simulink model "CoETS_TSEACo"  (R2016b)
settings: configuration reference "CodeGenConfigSet" (kept outside this file)
values from neighbouring files (symbols this model uses):
  CoETS_ctEngEmgcyRunCnt_C = Calibration.Parameter    [init_CoETS_TSEACo.m]
  CoETS_nTSCRmpSlopeNeg_C = Calibration.Parameter    [init_CoETS_TSEACo.m]
  CoETS_nTSCRmpSlopePos_C = Calibration.Parameter    [init_CoETS_TSEACo.m]
  CoETS_numTSEAPrioAE_C = Calibration.Parameter    [init_CoETS_TSEACo.m]
  CoETS_numTSEAPrioDE_C = Calibration.Parameter    [init_CoETS_TSEACo.m]
  CoETS_numTSEAPrioGpsLim_C = Calibration.Parameter    [init_CoETS_TSEACo.m]
  CoETS_numTSEAPrioPE_C = Calibration.Parameter    [init_CoETS_TSEACo.m]
  CoETS_numTSEAPrioTE_C = Calibration.Parameter    [init_CoETS_TSEACo.m]
  CoETS_numTSEAPrioVE_C = Calibration.Parameter    [init_CoETS_TSEACo.m]
  CoETS_stEngEmgcyRunEN_C = Calibration.Parameter    [init_CoETS_TSEACo.m]
  CoETS_stStartRelayCtrl_C = Calibration.Parameter    [init_CoETS_TSEACo.m]
  CoETS_stTboxUse_C = Calibration.Parameter    [init_CoETS_TSEACo.m]
  CoETS_stTSEATrqSpd_C = Calibration.Parameter    [init_CoETS_TSEACo.m]
  CoETS_swtTempSel_C = Calibration.Parameter    [init_CoETS_TSEACo.m]
  CoETS_tEngEmgcyRunTemp_C = Calibration.Parameter    [init_CoETS_TSEACo.m]
  CoETS_tiEngEmgcyRunTime_C = Calibration.Parameter    [init_CoETS_TSEACo.m]
  CoETS_tiEngEmgcyStartTime_C = Calibration.Parameter    [init_CoETS_TSEACo.m]
  CoETS_tiEngLockTime_C = Calibration.Parameter    [init_CoETS_TSEACo.m]
  CoETS_tiSetTimeTSEReq_CUR = Calibration.Parameter    [init_CoETS_TSEACo.m]
  CoETS_tiSetTimeTSEReq_CURX = Calibration.Parameter    [init_CoETS_TSEACo.m]
  CoETS_TrqTSCRmpSlopeNeg_C = Calibration.Parameter    [init_CoETS_TSEACo.m]
  CoETS_TrqTSCRmpSlopePos_C = Calibration.Parameter    [init_CoETS_TSEACo.m]
  Ecu_stGps_Status_C = Calibration.Parameter    [init_CoETS_TSEACo.m]
  EngPrt_nRateSp_C = Calibration.Parameter    [init_CoETS_TSEACo.m]
  Gps_nSpdLmt_C = Calibration.Parameter    [init_CoETS_TSEACo.m]
  TSC_nAEDes_C = Calibration.Parameter    [init_CoETS_TSEACo.m]
  TSC_nDEDes_C = Calibration.Parameter    [init_CoETS_TSEACo.m]
  TSC_nPEDes_C = Calibration.Parameter    [init_CoETS_TSEACo.m]
  TSC_nTEDes_C = Calibration.Parameter    [init_CoETS_TSEACo.m]
  TSC_nVEDes_C = Calibration.Parameter    [init_CoETS_TSEACo.m]
  TSC_rTrqAEDes_C = Calibration.Parameter    [init_CoETS_TSEACo.m]
  TSC_rTrqDEDes_C = Calibration.Parameter    [init_CoETS_TSEACo.m]
  TSC_rTrqPEDes_C = Calibration.Parameter    [init_CoETS_TSEACo.m]
  TSC_rTrqTEDes_C = Calibration.Parameter    [init_CoETS_TSEACo.m]
  TSC_rTrqVEDes_C = Calibration.Parameter    [init_CoETS_TSEACo.m]
  TSC_stAEErr_C = Calibration.Parameter    [init_CoETS_TSEACo.m]
  TSC_stAEMode_C = Calibration.Parameter    [init_CoETS_TSEACo.m]
  TSC_stDEErr_C = Calibration.Parameter    [init_CoETS_TSEACo.m]
  TSC_stDEMode_C = Calibration.Parameter    [init_CoETS_TSEACo.m]
  TSC_stModeBypassEN_C = Calibration.Parameter    [init_CoETS_TSEACo.m]
  TSC_stPEErr_C = Calibration.Parameter    [init_CoETS_TSEACo.m]
  TSC_stPEMode_C = Calibration.Parameter    [init_CoETS_TSEACo.m]
  TSC_stTEErr_C = Calibration.Parameter    [init_CoETS_TSEACo.m]
  TSC_stTEMode_C = Calibration.Parameter    [init_CoETS_TSEACo.m]
  TSC_stVEErr_C = Calibration.Parameter    [init_CoETS_TSEACo.m]
  TSC_stVEMode_C = Calibration.Parameter    [init_CoETS_TSEACo.m]
undefined symbols (not defined in the file or in its folder): CoETS_TSEACo_DT, EngState_conv, HLSDem_KpCorFac_MAPX, Switch_conv, TSC1_stSource_conv
libraries: simulink x82, CXLib x8
(part 2 of 2)

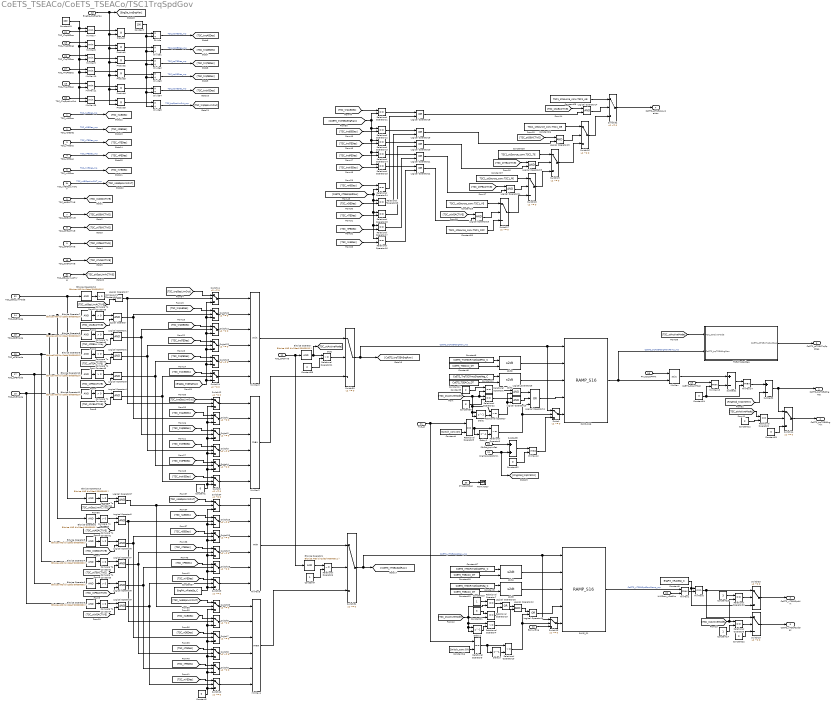
== system CoETS_TSEACo/CoETS_TSEACo/TSC1TrqSpdGov ==
  TSC_nAEDes : Inport  Tag=rpm  Description=Requested speed / speed limit by TSC1-AE message  OutMin=0  OutMax=6000  OutDataTypeStr=EngSpeed_rpm
  TSC_nDEDes : Inport  Tag=rpm  Description=|  Port=2  OutMin=0  OutMax=8000  OutDataTypeStr=EngSpeed_rpm
      | Requested speed / speed limit by TSC1-DE CAN
      | message rpm
  TSC_nTEDes : Inport  Tag=rpm  Description=|  Port=3  OutMin=0  OutMax=8000  OutDataTypeStr=EngSpeed_rpm
      | Requested speed / speed limit by TSC1-TE CAN
      | message rpm
  TSC_nPEDes : Inport  Tag=rpm  Description=|  Port=4  OutMin=0  OutMax=8000  OutDataTypeStr=EngSpeed_rpm
      | Requested speed / speed limit by TSC1-PE CAN
      | message rpm
  TSC_nVEDes : Inport  Tag=rpm  Description=|  Port=5  OutMin=0  OutMax=8000  OutDataTypeStr=EngSpeed_rpm
      | Requested speed / speed limit by TSC1-VE CAN
      | message rpm
  TSC_stAEACTIVE : Inport  Port=6
  TSC_stDEACTIVE : Inport  Port=7
  TSC_stTEACTIVE : Inport  Port=8
  TSC_stPEACTIVE : Inport  Port=9
  TSC_stVEACTIVE : Inport  Port=10
  TSC_stACTIVE : Inport  Port=11
  Epm_nEng : Inport  Tag=rpm  Description=Engine speed  Port=12  OutMin=0  OutMax=6000  OutDataTypeStr=EngSpeed_rpm
  PT_trqCrSPTPrt : Inport  Tag=Nm  Description=Application parameter for powertrain protection train protection torque(crankshaft torque)  Port=13  OutMin=-3000  OutMax=3000  OutDataTypeStr=Trq_Nm
  TSC_stAEMode : Inport  Description=Override control mode of TSC1-AE CAN message  Port=14  OutMin=0  OutMax=3  OutDataTypeStr=State_uint8
  TSC_stDEMode : Inport  Description=Override control mode of TSC1-DE CAN message  Port=15  OutMin=0  OutMax=3  OutDataTypeStr=State_uint8
  TSC_stTEMode : Inport  Description=Override control mode of TSC1-TE CAN message  Port=16  OutMin=0  OutMax=3  OutDataTypeStr=State_uint8
  TSC_stPEMode : Inport  Description=Override control mode of TSC1-PE CAN message  Port=17  OutMin=0  OutMax=3  OutDataTypeStr=State_uint8
  TSC_stVEMode : Inport  Description=Override control mode of TSC1-VE CAN message.  Port=18  OutMin=0  OutMax=3  OutDataTypeStr=State_uint8
  PthSet_trqInrSet : Inport  Port=19
  HLSDem_nSetPLo : Inport  Port=20
  T15_st : Inport  Port=21
  RngMod_trqCrSMin : Inport  Port=22
  EngDa_trqEngMax : Inport  Tag=Nm  Description=Maximum engine output torque  Port=23  OutMin=-3276.8  OutMax=3276.7  OutDataTypeStr=Trq_Nm
  TSC_rTrqAEDes : Inport  Description=|  Port=24  OutMin=0  OutMax=125  OutDataTypeStr=State_uint8
      | Requested torque percent / torque limit by TSC1-AE CAN
      | message Nm
  TSC_rTrqDEDes : Inport  Description=|  Port=25  OutMin=0  OutMax=125  OutDataTypeStr=State_uint8
      | Requested torque percent/ torque limit by TSC1-DE CAN
      | message Nm
  TSC_rTrqTEDes : Inport  Description=|  Port=26  OutMin=0  OutMax=125  OutDataTypeStr=State_uint8
      | Requested torque percent / torque limit by TSC1-TE CAN
      | message Nm
  TSC_rTrqPEDes : Inport  Description=|  Port=27  OutMin=0  OutMax=125  OutDataTypeStr=State_uint8
      | Requested torque percent/ torque limit by TSC1-PE CAN
      | message Nm
  TSC_rTrqVEDes : Inport  Description=|  Port=28  OutMin=0  OutMax=125  OutDataTypeStr=State_uint8
      | Requested torque percent/ torque limit by TSC1-VE CAN
      | message Nm
  CoETS_trqUnFltLtd : Inport  Port=29
  PT_trqCrSDes : Inport  Tag=Nm  Description=Application parameter for requested propulsion torque to engine(crankshaft torque)  Port=30
  TSC_stGpsLimACTIVE : Inport  Port=31
  TSC_stGpsLimMode : Inport  Description=Override control mode of TSC1-AE CAN message  Port=32  OutMin=0  OutMax=3  OutDataTypeStr=State_uint8
  TSC_rTrqGpsLimOut : Inport  Description=|  Port=33  OutMin=0  OutMax=125  OutDataTypeStr=State_uint8
      | Requested torque percent/ torque limit by TSC1-VE CAN
      | message Nm
  TSC_nAEGpsLimOUT : Inport  Tag=rpm  Description=Requested speed / speed limit by TSC1-AE message  Port=34  OutMin=0  OutMax=6000  OutDataTypeStr=EngSpeed_rpm
  Bitwise Operator : simulink/Logic and Bit Operations/Bitwise Operator  logicop=AND  UseBitMask=on  BitMask=bin2dec('00000011')  BitMaskRealWorld=Stored Integer
  Bitwise Operator1 : simulink/Logic and Bit Operations/Bitwise Operator  logicop=AND  UseBitMask=on  BitMask=bin2dec('00000011')  BitMaskRealWorld=Stored Integer
  Bitwise Operator{7..12} (6 alike) : simulink/Logic and Bit Operations/Bitwise Operator  logicop=AND  UseBitMask=on  BitMask=bin2dec('00000010')  BitMaskRealWorld=Stored Integer
  Bitwise Operator{2..6,13} (6 alike) : simulink/Logic and Bit Operations/Bitwise Operator  logicop=AND  UseBitMask=on  BitMask=bin2dec('00000001')  BitMaskRealWorld=Stored Integer
  Compare To Constant{,1..11} (12 alike) : simulink/Logic and Bit Operations/Compare To Constant  relop=>  const=0  OutDataTypeStr=boolean
  Constant : Constant  Value=100  OutDataTypeStr=Inherit: Inherit via back propagation
  Constant{1..2,22,24,31..32} (6 alike) : Constant  Value=0  OutDataTypeStr=Inherit: Inherit via back propagation
  Constant10 : Constant  Value=CoETS_TrqTSCRmpSlopeNeg_C
  Constant{8,11,13,18} (4 alike) : Constant  Value=CoETS_TSEACo_DT
  Constant12 : Constant  Value=2  OutDataTypeStr=Inherit: Inherit via back propagation
  Constant14 : Constant  OutDataTypeStr=Inherit: Inherit via back propagation
  Constant15 : Constant  OutDataTypeStr=Inherit: Inherit via back propagation
  Constant16 : Constant  Value=Switch_conv.ON
  Constant17 : Constant  Value=CoETS_nTSCRmpSlopePos_C
  Constant19 : Constant  Value=100  OutDataTypeStr=Inherit: Inherit via back propagation
  Constant20 : Constant  Value=TSC1_stSource_conv.TSC1_OFF
  Constant21 : Constant  Value=3  OutDataTypeStr=Inherit: Inherit via back propagation
  Constant23 : Constant  Value=3  OutDataTypeStr=Inherit: Inherit via back propagation
  Constant25 : Constant  Value=TSC1_stSource_conv.TSC1_AE
  Constant26 : Constant  Value=TSC1_stSource_conv.TSC1_DE
  Constant27 : Constant  Value=TSC1_stSource_conv.TSC1_PE
  Constant28 : Constant  Value=TSC1_stSource_conv.TSC1_TE
  Constant29 : Constant  Value=TSC1_stSource_conv.TSC1_VE
  Constant3 : Constant  Value=2  OutDataTypeStr=Inherit: Inherit via back propagation
  Constant30 : Constant  Value=3  OutDataTypeStr=Inherit: Inherit via back propagation
  Constant37 : Constant  Value=EngPrt_nRateSp_C
  Constant38 : Constant  Value=2  OutDataTypeStr=Inherit: Inherit via back propagation
  Constant4 : Constant  Value=Switch_conv.ON
  Constant5 : Constant  Value=CoETS_nTSCRmpSlopeNeg_C
  Constant6 : Constant  Value=CoETS_TrqTSCRmpSlopePos_C
  Constant7 : Constant  OutDataTypeStr=Inherit: Inherit via back propagation
  Constant9 : Constant  Value=EngPrt_nRateSp_C
  Delay : Delay  DelayLength=1  InitialConditionSource=Input port  InitialCondition=0
      settings: InputPortMap=u0,p4
  Delay1 : Delay  DelayLength=1  InitialCondition=0
  Delay2 : Delay  DelayLength=1  InitialConditionSource=Input port  InitialCondition=0
      settings: InputPortMap=u0,p4
  Delay3 : Delay  DelayLength=1  InitialCondition=0
  Divide{,1..5} (6 alike) : Product  Inputs=*/  OutDataTypeStr=Inherit: Inherit via back propagation  SaturateOnIntegerOverflow=on
  Logical Operator{,1..10,12,14..15,17,23..27} (20 alike) : Logic  AllPortsSameDT=off  OutDataTypeStr=boolean
  Logical Operator11 : Logic  Operator=OR  Inputs=3  AllPortsSameDT=off  OutDataTypeStr=boolean
  Logical Operator{13,16,18..22} (7 alike) : Logic  Operator=OR  AllPortsSameDT=off  OutDataTypeStr=boolean
  MinMax{,6..11,15} (8 alike) : MinMax  Inputs=2
  MinMax{1,12..14} (4 alike) : MinMax  Function=max  Inputs=2
  MinMax2 : MinMax  Function=max  Inputs=6
  MinMax3 : MinMax  Inputs=6
  MinMax4 : MinMax  Function=max  Inputs=6
  MinMax5 : MinMax  Inputs=6
  Product{,1..5} (6 alike) : Product  SaturateOnIntegerOverflow=on
  RAMP_S1 : CXLib/RAMP_S16
  RAMP_S16 : CXLib/RAMP_S16
  Relational Operator{,4..6,10,21} (6 alike) : RelationalOperator  Operator=~=  OutDataTypeStr=boolean  RndMeth=Simplest
  Relational Operator{1..3,7..9,11..20,22..24} (19 alike) : RelationalOperator  Operator===  OutDataTypeStr=boolean  RndMeth=Simplest
  Subtract1 : Sum  Inputs=+-  OutDataTypeStr=Inherit: Inherit via back propagation  SaturateOnIntegerOverflow=on  InputSameDT=on
  Subtract2 : Sum  Inputs=+-  OutDataTypeStr=Inherit: Inherit via back propagation  SaturateOnIntegerOverflow=on  InputSameDT=on
  Subtract3 : Sum  OutDataTypeStr=Inherit: Inherit via back propagation  SaturateOnIntegerOverflow=on  InputSameDT=on
  Switch{,1..35} (36 alike) : Switch  Criteria=u2 ~= 0
  TSEATrqSpdReq : Subsystem
  Terminator : Terminator
  s2dt{1..4} (4 alike) : CXLib/s2dt
  CoETS_trqTSEAEngMax : Outport
  CoETS_trqTSEAEngMin : Outport  Tag=Nm  Description=torque request to engine intervention increment(Min)  Port=2  OutMin=-3276  OutMax=3276  OutDataTypeStr=Trq_Nm
  CoETS_nTSEASpdLim : Outport  Port=3
  CoETS_stTSEASourceActv : Outport  Description=Identification name / number of the currently active EISGov client, which determines the current controller parameters  Port=4
  CoETS_nTSEASpdDes : Outport  Port=5
  CoETS_stTSEATrqSpdReq : Outport  Port=6
  wires:
  Switch30/1 -> [CoETS_trqTSEAEngRaw], RAMP_S16/1, Switch/1  "CoETS_trqTSEAEngRaw_mp"
  MinMax3/1 -> Switch30/1
  MinMax2/1 -> Switch30/3
  Constant38/1 -> Relational Operator21/2
  MinMax4/1 -> Switch31/3
  MinMax5/1 -> Switch31/1
  Relational Operator21/1 -> Switch30/2
  Bitwise Operator/1 -> Relational Operator21/1, [TSC_stActiveMode]
  [EngDa_trqEngMax] -> Switch11/3, Switch20/3, Switch21/3, Switch22/3, Switch23/3, Switch24/3
  Constant37/1 -> Switch25/3, Switch34/3, Switch26/3, Switch27/3, Switch28/3, Switch29/3
  Constant1/1 -> Switch4/3, Switch3/3, Switch2/3, Switch1/3, Switch12/3, Switch5/3
  Constant2/1 -> Switch35/3, Switch6/3, Switch7/3, Switch8/3, Switch9/3, Switch10/3
  Constant7/1 -> Relational Operator6/2
  Bitwise Operator1/1 -> Relational Operator6/1
  Relational Operator6/1 -> Switch31/2
  [TSC_stActiveMode] -> Relational Operator1/2, Relational Operator22/1, Relational Operator/1, Delay/2, Delay/1
  Delay/1 -> Relational Operator/2
  Compare To Constant5/1 -> Logical Operator/1
  TSC_stAEACTIVE/1 -> [TSC_stAEACTIVE]
  Compare To Constant6/1 -> Logical Operator1/1
  Compare To Constant7/1 -> Logical Operator2/1
  Logical Operator1/1 -> Switch2/2, Switch21/2
  Logical Operator2/1 -> Switch3/2, Switch22/2
  Compare To Constant8/1 -> Logical Operator3/1
  Logical Operator3/1 -> Switch4/2, Switch23/2
  Compare To Constant9/1 -> Logical Operator4/1
  Logical Operator4/1 -> Switch5/2, Switch24/2
  Logical Operator/1 -> Switch20/2, Switch1/2
  TSC_stAEMode/1 -> Bitwise Operator7/1, Bitwise Operator2/1
  Bitwise Operator2/1 -> Compare To Constant/1
  Bitwise Operator3/1 -> Compare To Constant1/1
  TSC_stDEMode/1 -> Bitwise Operator8/1, Bitwise Operator3/1
  Bitwise Operator4/1 -> Compare To Constant2/1
  TSC_stTEMode/1 -> Bitwise Operator9/1, Bitwise Operator4/1
  Bitwise Operator5/1 -> Compare To Constant3/1
  TSC_stPEMode/1 -> Bitwise Operator10/1, Bitwise Operator5/1
  Bitwise Operator6/1 -> Compare To Constant4/1
  TSC_stVEMode/1 -> Bitwise Operator11/1, Bitwise Operator6/1
  Bitwise Operator7/1 -> Compare To Constant5/1
  Bitwise Operator8/1 -> Compare To Constant6/1
  Bitwise Operator9/1 -> Compare To Constant7/1
  Bitwise Operator10/1 -> Compare To Constant8/1
  Bitwise Operator11/1 -> Compare To Constant9/1
  Compare To Constant/1 -> Logical Operator5/1
  TSC_stDEACTIVE/1 -> [TSC_stDEACTIVE]
  TSC_stTEACTIVE/1 -> [TSC_stTEACTIVE]
  TSC_stPEACTIVE/1 -> [TSC_stPEACTIVE]
  TSC_stVEACTIVE/1 -> [TSC_stVEACTIVE]
  [TSC_stAEACTIVE] -> Logical Operator/2
  [TSC_stDEACTIVE] -> Logical Operator1/2
  [TSC_stTEACTIVE] -> Logical Operator2/2
  [TSC_stPEACTIVE] -> Logical Operator3/2
  [TSC_stVEACTIVE] -> Logical Operator4/2
  [TSC_stAEACTIVE] -> Logical Operator5/2
  Logical Operator5/1 -> Switch6/2, Switch25/2
  Compare To Constant1/1 -> Logical Operator6/1
  [TSC_stDEACTIVE] -> Logical Operator6/2
  Logical Operator6/1 -> Switch7/2, Switch26/2
  Compare To Constant2/1 -> Logical Operator7/1
  [TSC_stTEACTIVE] -> Logical Operator7/2
  Compare To Constant3/1 -> Logical Operator8/1
  [TSC_stPEACTIVE] -> Logical Operator8/2
  Compare To Constant4/1 -> Logical Operator9/1
  [TSC_stVEACTIVE] -> Logical Operator9/2
  Logical Operator7/1 -> Switch8/2, Switch27/2
  Logical Operator8/1 -> Switch9/2, Switch28/2
  Logical Operator9/1 -> Switch10/2, Switch29/2
  Constant3/1 -> Relational Operator1/1
  Relational Operator/1 -> Logical Operator10/2, Logical Operator26/2
  RAMP_S16/1 -> TSEATrqSpdReq/2(CoETS_trqTSEAEngRaw), MinMax/2  "CoETS_trqTSEAEngRawRamp_mp"
  Constant8/1 -> s2dt2/2
  Constant6/1 -> s2dt2/1
  s2dt2/1 -> RAMP_S16/2
  Constant11/1 -> s2dt1/2
  Constant10/1 -> s2dt1/1
  s2dt1/1 -> RAMP_S16/3
  Switch14/1 -> CoETS_trqTSEAEngMin/1
  [TSC_stActiveMode] -> Relational Operator2/1
  Constant12/1 -> Relational Operator2/2
  Relational Operator2/1 -> Switch14/2
  Switch/1 -> RAMP_S16/5
  Logical Operator11/1 -> RAMP_S16/4
  Constant4/1 -> Relational Operator3/2
  Delay1/1 -> Relational Operator5/2
  Relational Operator3/1 -> Delay1/1, Relational Operator5/1
  Relational Operator5/1 -> Logical Operator11/3, Switch/2
  PT_trqCrSPTPrt/1 -> MinMax/1
  [TSC_stActiveMode] -> Relational Operator19/2, Delay2/2, Delay2/1, Relational Operator4/1, Relational Operator7/2
  Delay2/1 -> Relational Operator4/2
  Constant15/1 -> Relational Operator7/1
  Relational Operator4/1 -> Logical Operator12/2
  MinMax6/1 -> Switch33/1, Switch15/1
  Constant18/1 -> s2dt4/2
  Constant17/1 -> s2dt4/1
  s2dt4/1 -> RAMP_S1/2
  Constant13/1 -> s2dt3/2
  Constant5/1 -> s2dt3/1
  s2dt3/1 -> RAMP_S1/3
  Constant14/1 -> Relational Operator8/2
  Relational Operator8/1 -> Switch15/2
  Epm_nEng/1 -> Switch13/3
  Switch13/1 -> RAMP_S1/5
  Logical Operator12/1 -> Logical Operator13/1
  Logical Operator13/1 -> RAMP_S1/4
  T15_st/1 -> Relational Operator3/1, Relational Operator9/1
  Constant16/1 -> Relational Operator9/2
  Delay3/1 -> Relational Operator10/2
  Relational Operator9/1 -> Delay3/1, Relational Operator10/1
  Relational Operator10/1 -> Switch13/2, Logical Operator13/2
  Constant22/1 -> Switch15/3
  Constant25/1 -> Switch32/1
  Constant27/1 -> Switch18/1
  Constant28/1 -> Switch19/1
  Constant26/1 -> Switch16/1
  Constant20/1 -> Switch17/3
  Constant29/1 -> Switch17/1
  Switch17/1 -> Switch18/3
  Switch18/1 -> Switch19/3
  Switch19/1 -> Switch16/3
  Switch16/1 -> Switch32/3
  Switch32/1 -> CoETS_stTSEASourceActv/1
  [TSC_stAEACTIVE] -> Logical Operator14/1
  TSC_nAEDes/1 -> [TSC_nAEDes]  "TSC_nAEDes_mp"
  TSC_nDEDes/1 -> [TSC_nDEDes]  "TSC_nDEDes_mp"
  TSC_nTEDes/1 -> [TSC_nTEDes]  "TSC_nTEDes_mp"
  TSC_nPEDes/1 -> [TSC_nPEDes]  "TSC_nPEDes_mp"
  TSC_nVEDes/1 -> [TSC_nVEDes]  "TSC_nVEDes_mp"
  [TSC_trqAEDes] -> Switch20/1
  [TSC_trqAEDes] -> Switch1/1
  [TSC_trqDEDes] -> Switch21/1
  [TSC_trqDEDes] -> Switch2/1
  [TSC_trqTEDes] -> Switch22/1
  [TSC_trqTEDes] -> Switch3/1
  [TSC_trqPEDes] -> Switch23/1
  [TSC_trqPEDes] -> Switch4/1
  [TSC_trqVEDes] -> Switch24/1
  [TSC_trqVEDes] -> Switch5/1
  [TSC_nAEDes] -> Switch25/1
  [TSC_nAEDes] -> Switch6/1
  [TSC_nDEDes] -> Switch7/1
  [TSC_nDEDes] -> Switch26/1
  [TSC_nTEDes] -> Switch27/1
  [TSC_nTEDes] -> Switch8/1
  [TSC_nPEDes] -> Switch9/1
  [TSC_nVEDes] -> Switch10/1
  [TSC_nVEDes] -> Switch29/1
  [TSC_nPEDes] -> Switch28/1
  Logical Operator14/1 -> Switch32/2
  [TSC_stDEACTIVE] -> Logical Operator15/1
  [TSC_trqDEDes] -> Relational Operator12/2
  Logical Operator15/1 -> Switch16/2
  [TSC_trqAEDes] -> Relational Operator11/1
  [CoETS_trqTSEAEngRaw] -> Relational Operator11/2, Relational Operator15/1, Relational Operator14/1, Relational Operator13/1, Relational Operator12/1
  [TSC_trqTEDes] -> Relational Operator13/2
  [TSC_trqPEDes] -> Relational Operator14/2
  [TSC_trqVEDes] -> Relational Operator15/2
  Switch31/1 -> [CoETS_nTSEASpdRaw], RAMP_S1/1, Switch13/1  "CoETS_nTSEASpdRaw_mp"
  [TSC_nVEDes] -> Relational Operator16/2
  [TSC_nPEDes] -> Relational Operator17/2
  Constant21/1 -> Relational Operator19/1
  Relational Operator7/1 -> Logical Operator16/1
  Relational Operator19/1 -> Logical Operator16/2
  Logical Operator16/1 -> Logical Operator12/1
  Switch15/1 -> CoETS_nTSEASpdDes/1
  Switch33/1 -> CoETS_nTSEASpdLim/1
  [TSC_stActiveMode] -> Relational Operator20/2, Relational Operator8/1
  Relational Operator20/1 -> Switch33/2
  Constant23/1 -> Relational Operator20/1
  Constant30/1 -> Relational Operator22/2
  Constant31/1 -> Switch14/3
  [TSC_nTEDes] -> Relational Operator18/2
  Constant9/1 -> Switch33/3, MinMax6/1
  [TSC_nDEDes] -> Relational Operator23/2
  [TSC_nAEDes] -> Relational Operator24/1
  [CoETS_nTSEASpdRaw] -> Relational Operator16/1, Relational Operator17/1, Relational Operator18/1, Relational Operator23/1, Relational Operator24/2
  Relational Operator11/1 -> Logical Operator18/1
  Relational Operator24/1 -> Logical Operator18/2
  Relational Operator12/1 -> Logical Operator19/1
  Relational Operator23/1 -> Logical Operator19/2
  Relational Operator13/1 -> Logical Operator20/1
  Relational Operator18/1 -> Logical Operator20/2
  Relational Operator14/1 -> Logical Operator21/1
  Relational Operator17/1 -> Logical Operator21/2
  Relational Operator15/1 -> Logical Operator22/1
  Relational Operator16/1 -> Logical Operator22/2
  Logical Operator18/1 -> Logical Operator14/2
  Logical Operator19/1 -> Logical Operator15/2
  [TSC_stTEACTIVE] -> Logical Operator23/1
  Logical Operator23/1 -> Switch19/2
  Logical Operator20/1 -> Logical Operator23/2
  [TSC_stPEACTIVE] -> Logical Operator24/1
  Logical Operator24/1 -> Switch18/2
  Logical Operator21/1 -> Logical Operator24/2
  [TSC_stVEACTIVE] -> Logical Operator25/1
  Logical Operator25/1 -> Switch17/2
  Logical Operator22/1 -> Logical Operator25/2
  HLSDem_nSetPLo/1 -> MinMax1/2
  RAMP_S1/1 -> MinMax1/1  "CoETS_nTSEASpdRawRamp_mp"
  MinMax1/1 -> MinMax6/2
  EngDa_trqEngMax/1 -> Product5/2, Product4/2, Product3/2, Product2/2, Product1/2, Product/2, [EngDa_trqEngMax]
  Divide/1 -> [TSC_trqAEDes]  "TSC_trqAEDes_mp"
  Product1/1 -> Divide1/1
  Product/1 -> Divide/1
  Divide1/1 -> [TSC_trqDEDes]  "TSC_trqDEDes_mp"
  Product2/1 -> Divide2/1
  Divide2/1 -> [TSC_trqTEDes]  "TSC_trqTEDes_mp"
  Product3/1 -> Divide3/1
  Divide3/1 -> [TSC_trqPEDes]  "TSC_trqPEDes_mp"
  Product4/1 -> Divide4/1
  Divide4/1 -> [TSC_trqVEDes]  "TSC_trqVEDes_mp"
  Constant/1 -> Divide5/2, Divide4/2, Divide3/2, Divide2/2, Divide1/2, Divide/2
  Constant19/1 -> MinMax9/2, MinMax11/2, MinMax15/2, MinMax10/2, MinMax8/2, MinMax7/1
  MinMax7/1 -> Product/1
  TSC_rTrqAEDes/1 -> MinMax7/2
  MinMax8/1 -> Product1/1
  TSC_rTrqDEDes/1 -> MinMax8/1
  MinMax9/1 -> Product2/1
  TSC_rTrqTEDes/1 -> MinMax9/1
  MinMax10/1 -> Product3/1
  TSC_rTrqPEDes/1 -> MinMax10/1
  MinMax11/1 -> Product4/1
  TSC_rTrqVEDes/1 -> MinMax11/1
  Subtract2/1 -> Switch14/1, CoETS_trqTSEAEngMax/1
  TSEATrqSpdReq/1(CoETS_stTSEATrqSpdReq) -> CoETS_stTSEATrqSpdReq/1
  TSC_stACTIVE/1 -> Bitwise Operator1/1, Bitwise Operator/1
  Relational Operator22/1 -> Logical Operator10/1
  Relational Operator1/1 -> Logical Operator26/1
  Logical Operator10/1 -> Logical Operator11/2
  Logical Operator26/1 -> Logical Operator11/1
  MinMax13/1 -> Subtract1/2
  Constant24/1 -> MinMax14/2, MinMax13/2
  MinMax/1 -> Subtract1/1
  MinMax14/1 -> Subtract2/1
  Subtract1/1 -> MinMax14/1
  CoETS_trqUnFltLtd/1 -> MinMax13/1
  PT_trqCrSDes/1 -> Terminator/1
  PthSet_trqInrSet/1 -> Subtract3/1
  RngMod_trqCrSMin/1 -> [RngMod_trqCrSMin], Subtract3/2
  Subtract3/1 -> MinMax12/1
  Constant32/1 -> MinMax12/2
  MinMax12/1 -> Switch/3
  [RngMod_trqCrSMin] -> Subtract2/2
  TSC_stGpsLimACTIVE/1 -> [TSC_stGpsLimACTIVE]
  TSC_stGpsLimMode/1 -> Bitwise Operator13/1, Bitwise Operator12/1
  Compare To Constant10/1 -> Logical Operator17/1
  Bitwise Operator12/1 -> Compare To Constant10/1
  [TSC_stGpsLimACTIVE] -> Logical Operator17/2
  TSC_rTrqGpsLimOut/1 -> MinMax15/1
  MinMax15/1 -> Product5/1
  Product5/1 -> Divide5/1
  Divide5/1 -> [TSC_trqGpsLimOut]  "TSC_trqGpsLimOut_mp"
  Logical Operator17/1 -> Switch12/2, Switch11/2
  [TSC_trqGpsLimOut] -> Switch11/1
  Switch24/1 -> MinMax3/6
  Switch23/1 -> MinMax3/5
  Switch22/1 -> MinMax3/4
  Switch21/1 -> MinMax3/3
  Switch20/1 -> MinMax3/2
  Switch11/1 -> MinMax3/1
  Switch12/1 -> MinMax2/1
  [TSC_trqGpsLimOut] -> Switch12/1
  Switch5/1 -> MinMax2/6
  Switch4/1 -> MinMax2/5
  Switch3/1 -> MinMax2/4
  Switch2/1 -> MinMax2/3
  Switch1/1 -> MinMax2/2
  Bitwise Operator13/1 -> Compare To Constant11/1
  Compare To Constant11/1 -> Logical Operator27/1
  [TSC_stGpsLimACTIVE] -> Logical Operator27/2
  TSC_nAEGpsLimOUT/1 -> [TSC_nAEGpsLimOUT]  "TSC_nAEGpsLimOUT_mp"
  [TSC_nAEGpsLimOUT] -> Switch34/1
  Switch29/1 -> MinMax5/6
  Switch28/1 -> MinMax5/5
  Switch27/1 -> MinMax5/4
  Switch26/1 -> MinMax5/3
  Switch25/1 -> MinMax5/2
  Switch34/1 -> MinMax5/1
  Switch10/1 -> MinMax4/6
  Switch9/1 -> MinMax4/5
  Switch8/1 -> MinMax4/4
  Switch7/1 -> MinMax4/3
  Switch6/1 -> MinMax4/2
  Switch35/1 -> MinMax4/1
  Logical Operator27/1 -> Switch35/2, Switch34/2
  [TSC_nAEGpsLimOUT] -> Switch35/1
  [TSC_stActiveMode] -> TSEATrqSpdReq/1(TSC_stActiveMode)

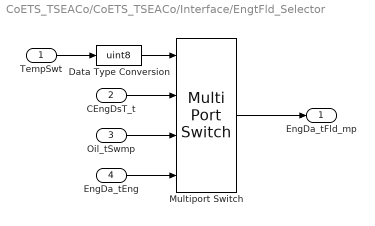
== system CoETS_TSEACo/CoETS_TSEACo/Interface/EngtFld_Selector ==
  TempSwt : Inport
  CEngDsT_t : Inport  Tag=deg  Description=engine coolant temperature after filter  Port=2
  Oil_tSwmp : Inport  Tag=deg  Description=Oil temperature in oil sump  Port=3
  EngDa_tEng : Inport  Tag=deg  Description=Engine temperature  Port=4
  Data Type Conversion : DataTypeConversion  OutDataTypeStr=uint8
  Multiport Switch : MultiPortSwitch  DataPortOrder=Zero-based contiguous
  EngDa_tFld_mp : Outport  Tag=deg  Description=Engine temperature field
  wires:
  CEngDsT_t/1 -> Multiport Switch/2
  Multiport Switch/1 -> EngDa_tFld_mp/1
  EngDa_tEng/1 -> Multiport Switch/4
  Oil_tSwmp/1 -> Multiport Switch/3
  Data Type Conversion/1 -> Multiport Switch/1
  TempSwt/1 -> Data Type Conversion/1

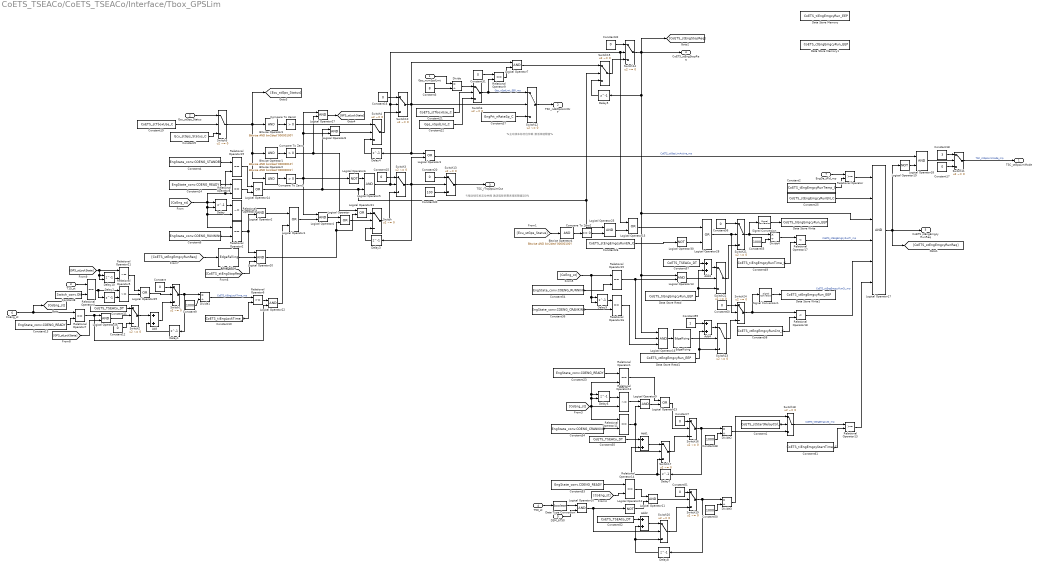
== system CoETS_TSEACo/CoETS_TSEACo/Interface/Tbox_GPSLim ==
  note: %被动锁车标志位仲裁 激活驾驶员需求扭矩限值到0%
  note: %主动锁车标志位仲裁 激活转速限值%
  Gps_numSpdLmt : Inport
  Ecu_stGps_Status : Inport  Port=2
  T15_st : Inport  Port=3
  T50_st : Inport  Port=4
  DSM_bT50 : Inport  Port=5
  CoEng_st : Inport  Port=6
  EngDa_tFld_mp : Inport  Port=7
  Add{,1..4} (5 alike) : Sum  SaturateOnIntegerOverflow=on  InputSameDT=on
  Bitwise Operator1 : simulink/Logic and Bit Operations/Bitwise Operator  logicop=AND  UseBitMask=on  BitMask=bin2dec('00000010')  BitMaskRealWorld=Stored Integer
  Bitwise Operator2 : simulink/Logic and Bit Operations/Bitwise Operator  logicop=AND  UseBitMask=on  BitMask=bin2dec('00000001')  BitMaskRealWorld=Stored Integer
  Bitwise Operator3 : simulink/Logic and Bit Operations/Bitwise Operator  logicop=AND  UseBitMask=on  BitMask=bin2dec('00000100')  BitMaskRealWorld=Stored Integer
  Bitwise Operator4 : simulink/Logic and Bit Operations/Bitwise Operator  logicop=AND  UseBitMask=on  BitMask=bin2dec('00000100')  BitMaskRealWorld=Stored Integer
  Compare To Zero : simulink/Logic and Bit Operations/Compare To Zero  relop=>  OutDataTypeStr=boolean
  Compare To Zero1 : simulink/Logic and Bit Operations/Compare To Zero  relop=>  OutDataTypeStr=boolean
  Compare To Zero2 : simulink/Logic and Bit Operations/Compare To Zero  relop===  OutDataTypeStr=boolean
  Compare To Zero3 : simulink/Logic and Bit Operations/Compare To Zero  relop=>  OutDataTypeStr=boolean
  Constant{,7,12,15..17,20,31..32,51,56,60} (12 alike) : Constant  Value=0  OutDataTypeStr=Inherit: Inherit via back propagation
  Constant1 : Constant  Value=CoETS_stStartRelayCtrl_C
  Constant10 : Constant  Value=CoETS_tiEngLockTime_C
  Constant{11,35,52,57} (4 alike) : Constant  Value=CoETS_TSEACo_DT
  Constant{13..14,23,53} (4 alike) : Constant  Value=EngState_conv.COENG_READY
  Constant18 : Constant  Value=3  OutDataTypeStr=Inherit: Inherit via back propagation
  Constant19 : Constant  Value=CoETS_stTboxUse_C
  Constant2 : Constant  Value=CoETS_tEngEmgcyRunTemp_C
  Constant21 : Constant  Value=CoETS_stTboxUse_C
  Constant22 : Constant  Value=Gps_nSpdLmt_C
  Constant25 : Constant  Value=CoETS_stEngEmgcyRunEN_C
  Constant26 : Constant  Value=CoETS_stEngEmgcyRunEN_C
  Constant3 : Constant  Value=8  OutDataTypeStr=Inherit: Inherit via back propagation
  Constant30 : Constant  Value=100  OutDataTypeStr=Inherit: Inherit via back propagation
  Constant34 : Constant  Value=EngState_conv.COENG_CRANKING
  Constant36 : Constant  Value=EngState_conv.COENG_CRANKING
  Constant37 : Constant  Value=EngPrt_nRateSp_C
  Constant4 : Constant  Value=EngState_conv.COENG_STANDBY
  Constant{9,48,50,55} (4 alike) : Constant  Value=1000  OutDataTypeStr=Inherit: Inherit via back propagation
  Constant49 : Constant  Value=CoETS_tiEngEmgcyRunTime_C
  Constant5 : Constant  Value=Ecu_stGps_Status_C
  Constant54 : Constant  Value=EngState_conv.COENG_RUNNING
  Constant58 : Constant  Value=CoETS_ctEngEmgcyRunCnt_C
  Constant59 : Constant  OutDataTypeStr=uint8
  Constant6 : Constant  Value=EngState_conv.COENG_RUNNING
  Constant61 : Constant  Value=CoETS_tiEngEmgcyStartTime_C
  Constant8 : Constant  Value=Switch_conv.ON
  Data Store Memory : DataStoreMemory  DataStoreName=CoETS_tiEngEmgcyRun_EEP  ReadBeforeWriteMsg=warning  WriteAfterWriteMsg=warning  WriteAfterReadMsg=warning  ShowAdditionalParam=off
  Data Store Memory1 : DataStoreMemory  DataStoreName=CoETS_ctEngEmgcyRun_EEP  ReadBeforeWriteMsg=warning  WriteAfterWriteMsg=warning  WriteAfterReadMsg=warning  ShowAdditionalParam=off
  Data Store Read : DataStoreRead  DataStoreName=CoETS_tiEngEmgcyRun_EEP
  Data Store Read1 : DataStoreRead  DataStoreName=CoETS_ctEngEmgcyRun_EEP
  Data Store Write : DataStoreWrite  DataStoreName=CoETS_tiEngEmgcyRun_EEP
  Data Store Write1 : DataStoreWrite  DataStoreName=CoETS_ctEngEmgcyRun_EEP
  Data Type Conversion : DataTypeConversion  OutDataTypeStr=boolean
  Delay{,6,9..10} (4 alike) : Delay  DelayLength=1  InitialConditionSource=Input port  InitialCondition=0
      settings: InputPortMap=u0,p4
  Delay{1..5,7..8} (7 alike) : Delay  DelayLength=1  InitialCondition=0
  Divide : Product  Inputs=*/  OutDataTypeStr=Inherit: Inherit via back propagation  InputSameDT=on
  Divide{1..4} (4 alike) : Product  Inputs=*/  OutDataTypeStr=Inherit: Inherit via back propagation
  EdgeFalling : CXLib/EdgeFalling
  EdgeRising : CXLib/EdgeRising
  Logical Operator{,1,3,14..15,21,23,28..29} (9 alike) : Logic  Operator=OR  AllPortsSameDT=off  OutDataTypeStr=boolean
  Logical Operator{2,4..5,7..11,13,18,22,25..27} (14 alike) : Logic  AllPortsSameDT=off  OutDataTypeStr=boolean
  Logical Operator{6,12,19,30} (4 alike) : Logic  Operator=NOT  AllPortsSameDT=off  OutDataTypeStr=boolean
  Logical Operator16 : Logic  Inputs=3  AllPortsSameDT=off  OutDataTypeStr=boolean
  Logical Operator17 : Logic  Inputs=6  AllPortsSameDT=off  OutDataTypeStr=boolean
  Logical Operator20 : Logic  Inputs=3  AllPortsSameDT=off  OutDataTypeStr=boolean
  Relational Operator : RelationalOperator  OutDataTypeStr=boolean  RndMeth=Simplest
  Relational Operator{1..2,7..8,11,14..16,19} (9 alike) : RelationalOperator  Operator===  OutDataTypeStr=boolean  RndMeth=Nearest  InputSameDT=on
  Relational Operator12 : RelationalOperator  Operator=~=  OutDataTypeStr=boolean  RndMeth=Nearest  InputSameDT=on
  Relational Operator13 : RelationalOperator  OutDataTypeStr=boolean  RndMeth=Simplest
  Relational Operator17 : RelationalOperator  Operator=<  OutDataTypeStr=boolean  RndMeth=Simplest  InputSameDT=on
  Relational Operator18 : RelationalOperator  Operator=<  OutDataTypeStr=boolean  RndMeth=Simplest
  Relational Operator21 : RelationalOperator  Operator=~=  OutDataTypeStr=boolean  RndMeth=Simplest
  Relational Operator3 : RelationalOperator  Operator=~=  OutDataTypeStr=boolean  RndMeth=Nearest  InputSameDT=on
  Relational Operator4 : RelationalOperator  Operator===  OutDataTypeStr=boolean  RndMeth=Simplest
  Relational Operator5 : RelationalOperator  Operator=~=  OutDataTypeStr=boolean  RndMeth=Simplest
  Relational Operator6 : RelationalOperator  OutDataTypeStr=boolean  RndMeth=Simplest  InputSameDT=on
  Relational Operator9 : RelationalOperator  Operator===  OutDataTypeStr=boolean  RndMeth=Simplest  InputSameDT=on
  Signal Conversion : SignalConversion  OverrideOpt=off
  Signal Conversion1 : SignalConversion  OverrideOpt=off
  Switch{,1..5,10..17,19..24} (20 alike) : Switch  Criteria=u2 ~= 0
  Switch18 : Switch  Criteria=u2 ~= 0  InputSameDT=on
  Switch6 : Switch  Criteria=u2 ~= 0  InputSameDT=on
  TSC_stGpsLimMode : Outport
  TSC_nAEGpsLimOUT : Outport  Port=2
  TSC_rTrqGpsLimOut : Outport  Port=3
  CoETS_stEngStopReq : Outport  Port=4
  CoETS_stEngEmgcyRunReq : Outport  Port=5
  wires:
  [CoEng_st] -> Relational Operator14/2
  Constant51/1 -> Switch19/1
  Constant50/1 -> Divide3/2
  Switch19/1 -> Delay8/1, Divide3/1
  Logical Operator10/1 -> Switch20/2, Logical Operator12/1
  Logical Operator11/1 -> Switch19/2
  Constant59/1 -> Add4/1
  Constant6/1 -> Relational Operator2/2
  Delay/1 -> Relational Operator3/1
  [CoEng_st] -> Relational Operator19/2, Relational Operator8/2, Relational Operator2/1, Relational Operator3/2, Delay/2, Delay/1
  Constant8/1 -> Relational Operator4/2
  Delay2/1 -> Relational Operator5/2
  Add/1 -> Switch1/3
  Divide1/1 -> Relational Operator6/1  "CoETS_tiEngLockTime_mp"
  Constant10/1 -> Relational Operator6/2
  Relational Operator4/1 -> Delay2/1, Relational Operator5/1
  CoEng_st/1 -> [CoEng_st], Relational Operator7/1
  Constant11/1 -> Switch2/1
  Delay1/1 -> Add/2
  Constant12/1 -> Switch2/3
  T15_st/1 -> Relational Operator4/1
  Constant/1 -> Switch1/1
  Constant9/1 -> Divide1/2
  Switch1/1 -> Divide1/1, Delay1/1
  Delay3/1 -> Switch/3
  Logical Operator1/1 -> Logical Operator4/2
  Constant14/1 -> Relational Operator8/1
  Bitwise Operator2/1 -> Compare To Zero1/1
  Constant16/1 -> Switch10/1
  Logical Operator6/1 -> Logical Operator5/1
  Delay4/1 -> Switch4/3
  Compare To Zero1/1 -> Logical Operator6/1, Logical Operator4/1, Logical Operator8/2, Logical Operator27/1
  Switch4/1 -> Switch10/3
  Switch10/1 -> Logical Operator7/1, Delay4/1, Logical Operator3/1, Switch12/2
  Constant15/1 -> Switch3/1
  Switch2/1 -> Add/1
  Constant13/1 -> Relational Operator7/2
  Bitwise Operator1/1 -> Compare To Zero/1
  Switch/1 -> Switch3/3
  Constant17/1 -> Switch11/3
  Constant30/1 -> Switch13/3
  Bitwise Operator3/1 -> Compare To Zero3/1
  Constant20/1 -> Switch13/1
  Switch13/1 -> TSC_rTrqGpsLimOut/1
  Constant31/1 -> Relational Operator9/1
  Constant18/1 -> Switch11/1
  Switch12/1 -> TSC_nAEGpsLimOUT/1
  Compare To Zero3/1 -> Switch4/1
  Relational Operator9/1 -> Logical Operator7/2
  Delay5/1 -> Switch15/3
  Switch15/1 -> Switch14/3
  Logical Operator2/1 -> Logical Operator1/1
  Constant32/1 -> Switch14/1
  Switch14/1 -> [CoETS_stEngStopReq], CoETS_stEngStopReq/1, Logical Operator17/3, Logical Operator13/1, Logical Operator16/1, Delay5/1
  Logical Operator7/1 -> Switch15/1
  Switch3/1 -> Switch13/2, Delay3/1, Logical Operator3/2
  Constant37/1 -> Switch12/3
  Logical Operator8/1 -> Switch4/2
  Relational Operator15/1 -> Logical Operator13/2, Logical Operator16/2
  Constant55/1 -> Divide4/2
  Logical Operator5/1 -> Logical Operator15/1, Switch14/2, Switch10/2, Switch3/2
  Logical Operator13/1 -> Switch22/2
  Divide4/1 -> Relational Operator17/1
  Constant56/1 -> Switch21/1
  Switch21/1 -> Signal Conversion/1, Divide4/1
  Relational Operator3/1 -> Logical Operator2/1
  Delay6/1 -> Relational Operator12/1
  Constant7/1 -> Switch16/1
  Relational Operator11/1 -> Switch17/2, Logical Operator9/2
  Switch16/1 -> Delay7/1, Divide2/1
  Constant48/1 -> Divide2/2
  [CoEng_st] -> Relational Operator11/1, Relational Operator12/2, Relational Operator1/2, Delay6/1, Delay6/2
  Relational Operator12/1 -> Logical Operator9/1
  Relational Operator2/1 -> Logical Operator20/1, Logical Operator2/2
  Constant34/1 -> Relational Operator11/2
  Switch11/1 -> TSC_stGpsLimMode/1  "TSC_stGpsLimMode_mp"
  Constant49/1 -> Relational Operator17/2
  Constant58/1 -> Relational Operator18/2
  Switch24/1 -> Relational Operator18/1, Signal Conversion1/1
  Data Store Read/1 -> Add3/2, Switch22/3
  Switch23/1 -> Switch24/3
  Add1/1 -> Switch17/1
  Switch18/1 -> Relational Operator13/1  "CoETS_tiEngEmgcySt_mp"
  T50_st/1 -> Data Type Conversion/1
  Data Type Conversion/1 -> Logical Operator10/1
  DSM_bT50/1 -> Logical Operator10/2
  Constant1/1 -> Switch18/2
  Constant54/1 -> Relational Operator15/2
  [CoEng_st] -> Relational Operator15/1, Delay9/1, Delay9/2
  Switch20/1 -> Switch19/3
  Constant36/1 -> Relational Operator16/2
  Logical Operator16/1 -> EdgeRising/1
  Constant53/1 -> Relational Operator14/1
  Logical Operator12/1 -> Logical Operator11/2
  Relational Operator14/1 -> Logical Operator11/1
  Constant61/1 -> Relational Operator13/2
  Delay8/1 -> Switch20/3, Add2/2
  Add2/1 -> Switch20/1
  Switch22/1 -> Switch21/3
  Add3/1 -> Switch22/1
  Delay7/1 -> Switch17/3, Add1/2
  Data Store Read1/1 -> Add4/2, Switch23/3
  Constant60/1 -> Switch24/1
  Delay9/1 -> Relational Operator16/1
  Signal Conversion1/1 -> Data Store Write1/1
  EdgeRising/1 -> Switch23/2
  Add4/1 -> Switch23/1
  Constant57/1 -> Add3/1
  Switch17/1 -> Switch16/3
  Constant52/1 -> Add2/1
  Logical Operator17/1 -> Logical Operator19/1, CoETS_stEngEmgcyRunReq/1, [CoETS_stEngEmgcyRunReq]
  Logical Operator18/1 -> Switch11/2
  Constant35/1 -> Add1/1
  Relational Operator16/1 -> Logical Operator16/3
  Signal Conversion/1 -> Data Store Write/1
  EngDa_tFld_mp/1 -> Relational Operator/1
  Constant2/1 -> Relational Operator/2
  Relational Operator/1 -> Logical Operator17/1
  Constant3/1 -> Divide/2
  Gps_numSpdLmt/1 -> Divide/1
  Divide3/1 -> Switch18/1
  Divide2/1 -> Switch18/3
  Switch5/1 -> [Ecu_stGps_Status], Bitwise Operator2/1, Bitwise Operator1/1, Bitwise Operator3/1
  Ecu_stGps_Status/1 -> Switch5/1
  Constant5/1 -> Switch5/3
  Constant19/1 -> Switch5/2
  [CoETS_stEngEmgcyRunReq] -> EdgeFalling/1
  EdgeFalling/1 -> Logical Operator20/2
  Logical Operator4/1 -> Logical Operator/1
  Logical Operator/1 -> Switch/2
  Logical Operator20/1 -> Logical Operator21/2, Logical Operator/2
  Logical Operator21/1 -> Switch/1
  [CoETS_stEngStopReq] -> Logical Operator20/3
  Divide/1 -> Switch6/1
  Switch6/1 -> Switch12/1, Relational Operator9/2  "Gps_nSpdLmt_EEP_mp"
  Constant21/1 -> Switch6/2
  Constant22/1 -> Switch6/3
  Relational Operator6/1 -> Logical Operator22/1
  Constant23/1 -> Relational Operator1/1
  Relational Operator1/1 -> Logical Operator23/1
  Logical Operator9/1 -> Logical Operator23/2
  Logical Operator23/1 -> Switch16/2
  Logical Operator19/1 -> Logical Operator18/2
  Logical Operator3/1 -> Logical Operator18/1  "CoETS_stGpsLimActive_mp"
  Constant4/1 -> Relational Operator19/1
  Relational Operator8/1 -> Logical Operator14/2
  Relational Operator19/1 -> Logical Operator14/1
  Logical Operator14/1 -> Logical Operator8/1, Logical Operator25/1, Switch15/2, Logical Operator5/2
  Logical Operator22/1 -> Logical Operator1/2
  [Ecu_stGps_Status] -> Bitwise Operator4/1
  Bitwise Operator4/1 -> Compare To Zero2/1
  Compare To Zero2/1 -> Logical Operator25/2
  Compare To Zero/1 -> Logical Operator27/2, Logical Operator21/1
  Logical Operator27/1 -> [GPS_stLockState]
  Relational Operator7/1 -> Logical Operator26/1, Logical Operator22/2
  Relational Operator5/1 -> Logical Operator29/2
  Logical Operator29/1 -> Switch1/2
  Logical Operator26/1 -> Switch2/2
  [GPS_stLockState] -> Logical Operator26/2
  Delay10/1 -> Relational Operator21/2
  [GPS_stLockState] -> Relational Operator21/1, Delay10/1, Delay10/2
  Relational Operator21/1 -> Logical Operator29/1
  Relational Operator13/1 -> Logical Operator17/6
  Relational Operator18/1 -> Logical Operator17/5  "CoETS_stEngEmgcyRunCt_mp"
  Relational Operator17/1 -> Logical Operator17/4  "CoETS_stEngEmgcyRunTi_mp"
  Constant25/1 -> Logical Operator17/2
  Logical Operator25/1 -> Logical Operator15/2
  Logical Operator15/1 -> Logical Operator28/1
  Logical Operator28/1 -> Switch24/2, Switch21/2
  Constant26/1 -> Logical Operator30/1
  Logical Operator30/1 -> Logical Operator28/2

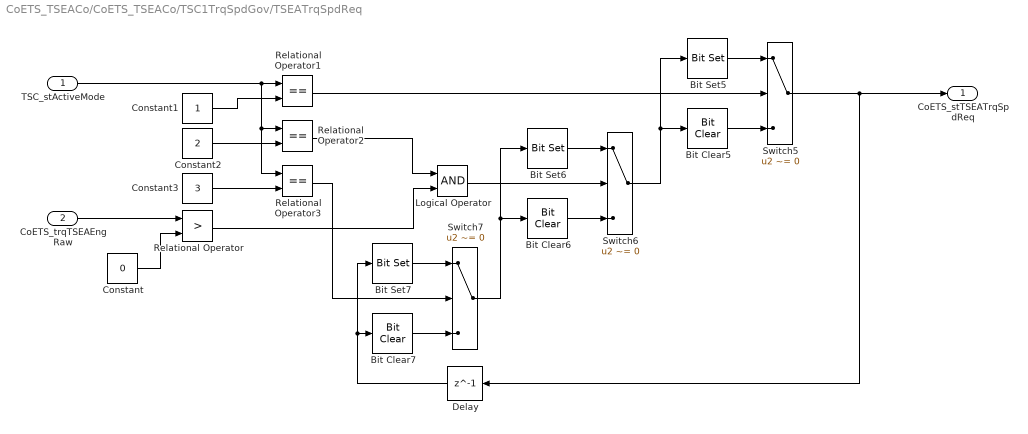
== system CoETS_TSEACo/CoETS_TSEACo/TSC1TrqSpdGov/TSEATrqSpdReq ==
  TSC_stActiveMode : Inport
  CoETS_trqTSEAEngRaw : Inport  Port=2
  Bit Clear5 : simulink/Logic and Bit Operations/Bit Clear  iBit=11
  Bit Clear6 : simulink/Logic and Bit Operations/Bit Clear  iBit=3
  Bit Clear7 : simulink/Logic and Bit Operations/Bit Clear  iBit=2
  Bit Set5 : simulink/Logic and Bit Operations/Bit Set  iBit=11
  Bit Set6 : simulink/Logic and Bit Operations/Bit Set  iBit=3
  Bit Set7 : simulink/Logic and Bit Operations/Bit Set  iBit=2
  Constant : Constant  Value=0  OutDataTypeStr=Inherit: Inherit via back propagation
  Constant1 : Constant  OutDataTypeStr=Inherit: Inherit via back propagation
  Constant2 : Constant  Value=2  OutDataTypeStr=Inherit: Inherit via back propagation
  Constant3 : Constant  Value=3  OutDataTypeStr=Inherit: Inherit via back propagation
  Delay : Delay  DelayLength=1  InitialCondition=0
  Logical Operator : Logic  AllPortsSameDT=off  OutDataTypeStr=boolean
  Relational Operator : RelationalOperator  Operator=>  OutDataTypeStr=boolean  RndMeth=Simplest  InputSameDT=on
  Relational Operator1 : RelationalOperator  Operator===  OutDataTypeStr=boolean  RndMeth=Simplest
  Relational Operator2 : RelationalOperator  Operator===  OutDataTypeStr=boolean  RndMeth=Simplest
  Relational Operator3 : RelationalOperator  Operator===  OutDataTypeStr=boolean  RndMeth=Simplest
  Switch5 : Switch  Criteria=u2 ~= 0
  Switch6 : Switch  Criteria=u2 ~= 0
  Switch7 : Switch  Criteria=u2 ~= 0
  CoETS_stTSEATrqSpdReq : Outport
  wires:
  Switch5/1 -> CoETS_stTSEATrqSpdReq/1, Delay/1
  Relational Operator1/1 -> Switch5/2
  Delay/1 -> Bit Set7/1, Bit Clear7/1
  Bit Set6/1 -> Switch6/1
  Bit Clear6/1 -> Switch6/3
  Constant2/1 -> Relational Operator2/2
  Constant3/1 -> Relational Operator3/2
  Constant1/1 -> Relational Operator1/2
  Switch6/1 -> Bit Clear5/1, Bit Set5/1
  Bit Clear5/1 -> Switch5/3
  Switch7/1 -> Bit Set6/1, Bit Clear6/1
  Bit Set5/1 -> Switch5/1
  TSC_stActiveMode/1 -> Relational Operator3/1, Relational Operator2/1, Relational Operator1/1
  Relational Operator3/1 -> Switch7/2
  Bit Set7/1 -> Switch7/1
  Bit Clear7/1 -> Switch7/3
  CoETS_trqTSEAEngRaw/1 -> Relational Operator/1
  Relational Operator2/1 -> Logical Operator/1
  Relational Operator/1 -> Logical Operator/2
  Logical Operator/1 -> Switch6/2
  Constant/1 -> Relational Operator/2
